simulink library "plant_lib"  (R2022b)
settings: Solver=VariableStepAuto  StartTime=0.0  StopTime=10.0  RelTol=1e-3
libraries: AMK_model_lib x1, battery_model_lib x1, driver_model_lib x1
settings Model: Creator=dr_pa  LastModifiedBy=dr_pa

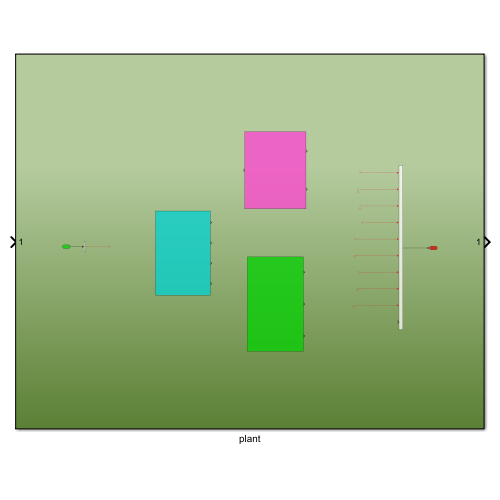
[thumbnail: Simulink's stored preview of the top-level diagram]
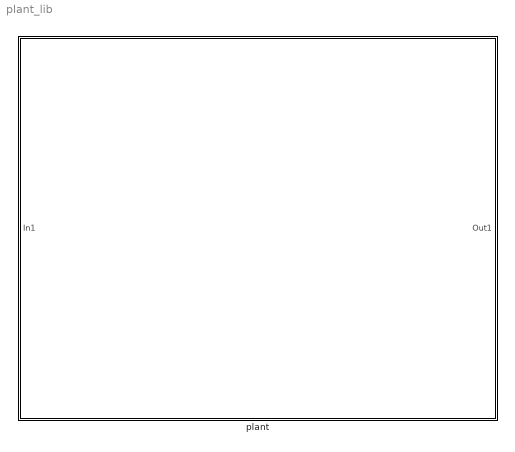
== system plant_lib ==
  plant : Subsystem

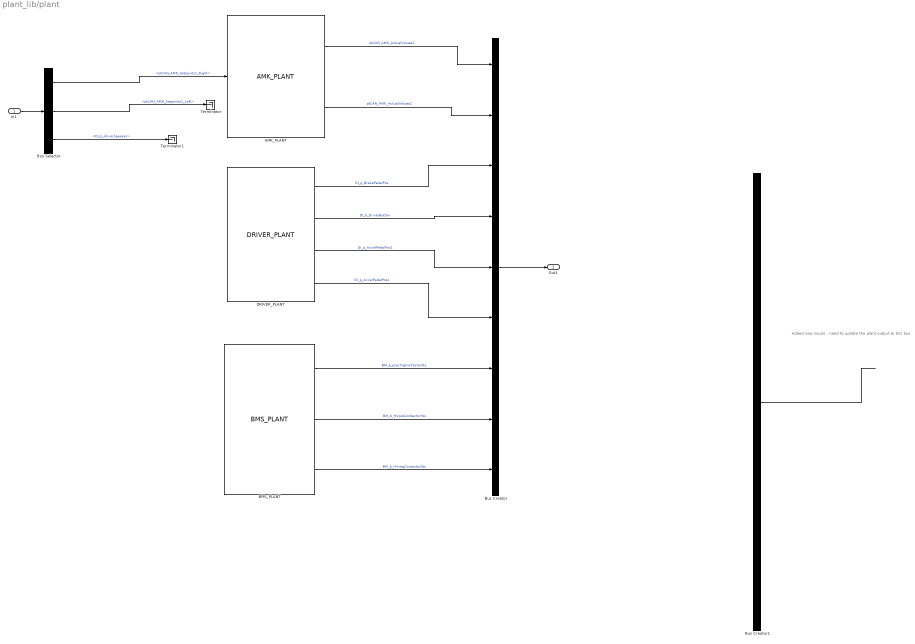
== system plant_lib/plant ==
  note: Added new inputs - need to update the plant output to this bus
  In1 : Inport
  AMK_PLANT : AMK_model_lib/AMK_PLANT  SystemSampleTime=-1  VariantActivationTime=update diagram  Latency=0  AutoFrameSizeCalculation=off
  BMS_PLANT : battery_model_lib/BMS_PLANT  SystemSampleTime=-1  VariantActivationTime=update diagram  Latency=0  AutoFrameSizeCalculation=off
  Bus Creator : BusCreator  Inputs=9
  Bus Creator1 : BusCreator  Inputs=12
  Bus Selector : BusSelector  OutputSignals=ptCAN_AMK_Setpoints1_Right,ptCAN_AMK_Setpoints1_Left,DI_b_driverSpeaker
  DRIVER_PLANT : driver_model_lib/DRIVER_PLANT  SystemSampleTime=-1  VariantActivationTime=update diagram  Latency=0  AutoFrameSizeCalculation=off
  Terminator : Terminator
  Terminator1 : Terminator
  Out1 : Outport
  wires:
  Bus Creator/1 -> Out1/1
  AMK_PLANT/1 -> Bus Creator/1  "ptCAN_AMK_ActualValues1"
  AMK_PLANT/2 -> Bus Creator/2  "ptCAN_AMK_ActualValues2"
  DRIVER_PLANT/1 -> Bus Creator/3  "DI_p_BrakePedalPos"
  DRIVER_PLANT/2 -> Bus Creator/4  "DI_b_DriverButton"
  DRIVER_PLANT/3 -> Bus Creator/5  "DI_p_AccelPedalPos1"
  DRIVER_PLANT/4 -> Bus Creator/6  "DI_p_AccelPedalPos2"
  BMS_PLANT/1 -> Bus Creator/7  "BM_b_prechrgContactorSts"
  BMS_PLANT/2 -> Bus Creator/8  "BM_b_HVposContactorSts"
  BMS_PLANT/3 -> Bus Creator/9  "BM_b_HVnegContactorSts"
  Bus Selector/1 -> AMK_PLANT/1  "<ptCAN_AMK_Setpoints1_Right>"
  ? -> Bus Creator1/6  "DI_V_BrakePedalPos"
  ? -> Bus Creator1/2  "ptCAN_AMK_ActualValues2_Right"
  ? -> Bus Creator1/12  "BM_b_HVnegContactorSts"
  ? -> Bus Creator1/4  "ptCAN_AMK_ActualValues2_Left"
  Bus Creator1/1 -> ?
  ? -> Bus Creator1/1  "ptCAN_AMK_ActualValues1_Right"
  ? -> Bus Creator1/5  "DI_V_SteeringAngle"
  ? -> Bus Creator1/11  "BM_b_HVposContactorSts"
  ? -> Bus Creator1/7  "DI_b_DriverButton"
  ? -> Bus Creator1/9  "DI_V_AccelPedalPos2"
  ? -> Bus Creator1/8  "DI_V_AccelPedalPos1"
  ? -> Bus Creator1/10  "BM_b_prechrgContactorSts"
  ? -> Bus Creator1/3  "ptCAN_AMK_ActualValues1_Left"
  Bus Selector/2 -> Terminator/1  "<ptCAN_AMK_Setpoints1_Left>"
  Bus Selector/3 -> Terminator1/1  "<DI_b_driverSpeaker>"
  In1/1 -> Bus Selector/1
